simulink model "tension"  (Simulink 3.00)
settings: Solver=ode45  SolverMode=SingleTasking  StartTime=0.0  StopTime=999999  MaxStep=10  RelTol=1e-3  AbsTol=1e-3
values from neighbouring files (symbols this model uses):
  b = 5E-5    (= 5e-05)    [Constants.m]
  J = 1    [Constants.m]
  Ka = 20    [Constants.m]
  Ke = 1.356    [Constants.m]
  Km = 1.36    [Constants.m]
  Kt = 0.0955    [Constants.m]
  R = 0.37    [Constants.m]
undefined symbols (not defined in the file or in its folder): L
settings Model: SaveTime=off  SaveOutput=off

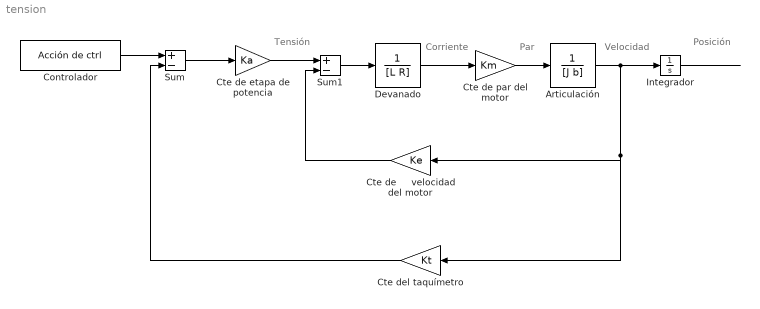
== system tension ==
  note: Tensión
  note: Corriente
  note: Par
  note: Velocidad
  note: Posición
  Articulación : TransferFcn  Numerator=[1]  Denominator=[J b]
  Controlador : FromFile  FileName=Acción de ctrl  SampleTime=0.001
  Cte de etapa de potencia : Gain  Gain=Ka  SaturateOnIntegerOverflow=on
  Cte de par del motor : Gain  Gain=Km  SaturateOnIntegerOverflow=on
  Cte de     velocidad del motor : Gain  Orientation=left  Gain=Ke  SaturateOnIntegerOverflow=on
  Cte del taquímetro : Gain  Orientation=left  Gain=Kt  SaturateOnIntegerOverflow=on
  Devanado : TransferFcn  Numerator=[1]  Denominator=[L R]
  Integrador : Integrator  ExternalReset=none  InitialConditionSource=internal  InitialCondition=0  LimitOutput=off  UpperSaturationLimit=inf  LowerSaturationLimit=-inf  ShowSaturationPort=off  ShowStatePort=off  AbsoluteTolerance=auto
  Sum : Sum  Inputs=+-  SaturateOnIntegerOverflow=on
  Sum1 : Sum  Inputs=+-  SaturateOnIntegerOverflow=on
  wires:
  Controlador/1 -> Sum/1
  Sum/1 -> Cte de etapa de potencia/1
  Sum1/1 -> Devanado/1
  Devanado/1 -> Cte de par del motor/1
  Cte de etapa de potencia/1 -> Sum1/1
  Cte de par del motor/1 -> Articulación/1
  Integrador/1 -> ?
  Articulación/1 -> Integrador/1, Cte de     velocidad del motor/1, Cte del taquímetro/1
  Cte de     velocidad del motor/1 -> Sum1/2
  Cte del taquímetro/1 -> Sum/2
